simulink library "flux_model_lib"  (R2015b)
settings: Solver=VariableStepAuto  StartTime=0.0  StopTime=10.0  RelTol=1e-3
undefined symbols (not defined in the file or in its folder): Lm, Lr, Rr
libraries: transformations_lib x2, simulink_extras x1
settings Model: Creator=zachn  LastModifiedBy=zachn

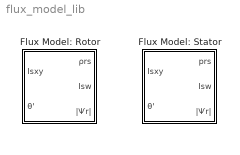
== system flux_model_lib ==
  Flux Model: Rotor : Subsystem  mask{Lm=1, Lr=1.1, Rr=1.1, dflx0=0}
      mask prompts: Lm "Mutual Inductance (H)"; Lr "Rotor Inductance (H)"; Rr "Rotor Resistance (Ω)"; dflx0 "Initial Rotor Flux"
      mask DialogControl DescGroupVar Prompt: SJSU EE37
      mask DialogControl DescTextVar Prompt: ACIM flux model expressed in the rotor frame
      mask DialogControl Container5 Prompt: Main
  Flux Model: Stator : Subsystem  mask{Lr=Lr, Lm=Lm, Rr=Rr, flux0=0.7}
      mask prompts: Lr "Rotor Inductance (Lr)"; Lm "Mutual Inductance (Lm)"; Rr "Rotor Resistance (Rr)"; flux0 "Initial Rotor Flux"
      mask DialogControl DescTextVar Prompt: ACIM flux model expressed in the stator frame

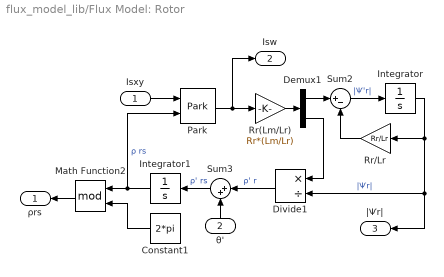
== system flux_model_lib/Flux Model: Rotor ==
  Isxy : Inport
  "θ' " : Inport  Port=2
  Constant1 : Constant  Value=2*pi
  Demux1 : Demux  Outputs=2
  Divide1 : Product  Inputs=*/
  Integrator : Integrator  InitialCondition=dflx0
  Integrator1 : Integrator
  Math Function2 : Math  Operator=mod  SaturateOnIntegerOverflow=on
  Park : transformations_lib/Park  IsInverse=on
  Rr(Lm/Lr) : Gain  Gain=Rr*(Lm/Lr)
  Rr/Lr : Gain  Gain=Rr/Lr
  Sum2 : Sum  Inputs=|+-
  Sum3 : Sum  Inputs=|++
  ρrs : Outport
  Isw : Outport  Port=2
  |Ѱr| : Outport  Port=3
  wires:
  Park/1 -> Rr(Lm/Lr)/1, Isw/1
  Rr(Lm/Lr)/1 -> Demux1/1
  Sum2/1 -> Integrator/1  "|Ѱ'r|"
  Integrator/1 -> |Ѱr|/1, Divide1/2, Rr/Lr/1  "|Ѱr|"
  Demux1/2 -> Divide1/1
  Divide1/1 -> Sum3/1  "ρ' r"
  Sum3/1 -> Integrator1/1  "ρ' rs"
  Integrator1/1 -> Math Function2/1, Park/2  "ρ rs"
  Isxy/1 -> Park/1
  "θ' "/1 -> Sum3/2
  Demux1/1 -> Sum2/1
  Rr/Lr/1 -> Sum2/2
  Constant1/1 -> Math Function2/2
  Math Function2/1 -> ρrs/1

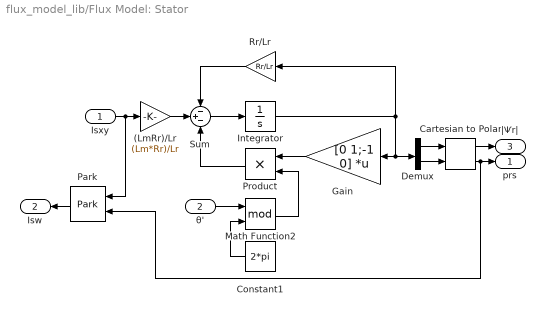
== system flux_model_lib/Flux Model: Stator ==
  Isxy : Inport
  θ' : Inport  Port=2
  (LmRr)/Lr : Gain  Gain=(Lm*Rr)/Lr
  Cartesian to Polar : simulink_extras/Transformations/Cartesian to Polar
  Constant1 : Constant  Value=2*pi
  Demux : Demux  Outputs=2
  Gain : Gain  Gain=[0 1;-1 0]  Multiplication=Matrix(K*u)
  Integrator : Integrator  InitialCondition=[flux0;flux0]
  Math Function2 : Math  Operator=mod  SaturateOnIntegerOverflow=on
  Park : transformations_lib/Park  IsInverse=on
  Product : Product
  Rr/Lr : Gain  Gain=Rr/Lr
  Sum : Sum  Inputs=-+-
  prs : Outport
  Isw : Outport  Port=2
  |Ѱr| : Outport  Port=3
  wires:
  Rr/Lr/1 -> Sum/1
  Isxy/1 -> Park/1, (LmRr)/Lr/1
  (LmRr)/Lr/1 -> Sum/2
  Sum/1 -> Integrator/1
  Product/1 -> Sum/3
  Gain/1 -> Product/1
  Cartesian to Polar/1 -> |Ѱr|/1
  Cartesian to Polar/2 -> Park/2, prs/1
  θ'/1 -> Math Function2/1
  Math Function2/1 -> Product/2
  Constant1/1 -> Math Function2/2
  Integrator/1 -> Rr/Lr/1, Demux/1, Gain/1
  Demux/1 -> Cartesian to Polar/1
  Demux/2 -> Cartesian to Polar/2
  Park/1 -> Isw/1
